simulink model "L400_airframe"  (R2024b)
settings: Solver=FixedStepAuto  StartTime=0  StopTime=10  FixedStep=5/1000  RelTol=1e-3
values from neighbouring files (symbols this model uses):
  db =     [L400_airframe_data.mat]
undefined symbols (not defined in the file or in its folder): lambda
libraries: aerolibconvert2 x16, simulink x6, matrix_library x4, aerolibactuator x2, shared6dof x1, aerolibtransform2 x1
(part 4 of 4)

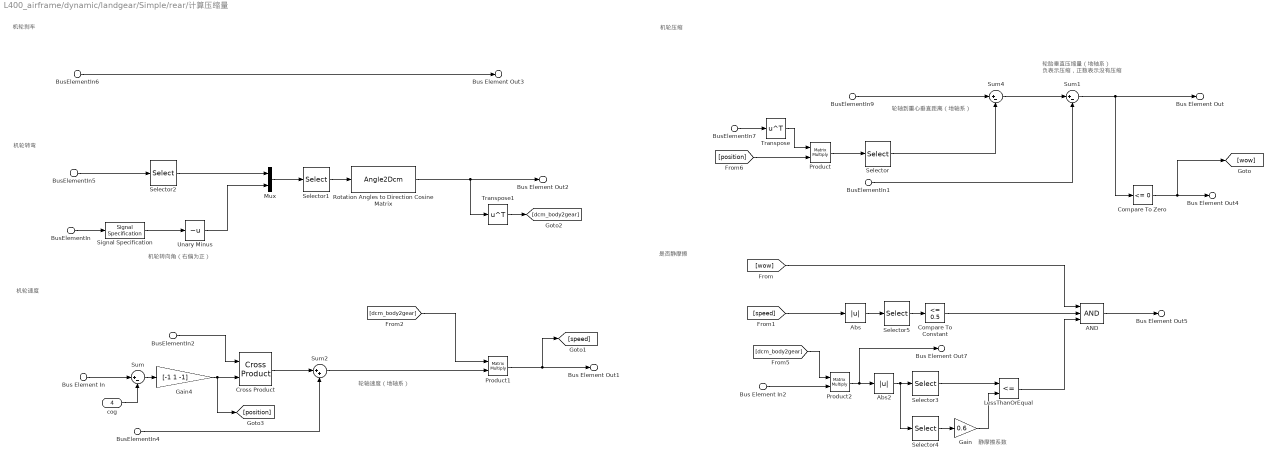
== system L400_airframe/dynamic/landgear/Simple/rear/计算压缩量 ==
  note: 静摩擦系数
  note: 机轮刹车
  note: 是否静摩擦
  note: 机轮速度
  note: 机轮转弯
  note: 机轮压缩
  note: 机轮转向角（右偏为正）
  note: 轮胎垂直压缩量（地轴系）
      | 负表示压缩，正数表示没有压缩
  note: 轮轴到重心垂直距离（地轴系）
  note: 轮轴速度（地轴系）
  BusElementIn : Inport  PortName=cmd  Element=DWheel
  BusElementIn6 : Inport  PortName=cmd  Element=DBrake
  BusElementIn7 : Inport  Port=2  PortName=state  Element=aircraft.attitude.Rbe
  BusElementIn2 : Inport  Port=2  PortName=state  Element=aircraft.attitude.p_q_r
  BusElementIn5 : Inport  Port=2  PortName=state  Element=aircraft.attitude.phi_theta_psi
  BusElementIn4 : Inport  Port=2  PortName=state  Element=aircraft.position.vx_vy_vz
  BusElementIn9 : Inport  Port=2  PortName=state  Element=aircraft.position.alt
  BusElementIn1 : Inport  Port=2  PortName=state  Element=environ.terrain.hground
  Bus Element In : Inport  Port=3  PortName=param  Element=position
  Bus Element In2 : Inport  Port=3  PortName=param  Element=reaction
  cog : Inport  Port=4
  AND : Logic  Inputs=3  IconShape=distinctive  AllPortsSameDT=off  OutDataTypeStr=boolean
  Abs : Abs  SaturateOnIntegerOverflow=off
  Abs2 : Abs  SaturateOnIntegerOverflow=off
  Compare To Constant : simulink/Logic and Bit Operations/Compare To Constant  relop=<=  const=0.5  OutDataTypeStr=boolean
  Compare To Zero : simulink/Logic and Bit Operations/Compare To Zero  relop=<=  OutDataTypeStr=boolean
  Cross Product : matrix_library/Cross Product
  Gain : Gain  Gain=0.6
  Gain4 : Gain  Gain=[-1 1 -1]
  LessThanOrEqual : RelationalOperator  Operator=<=  OutDataTypeStr=boolean  RndMeth=Simplest  InputSameDT=off
  Mux : Mux  Inputs=2
  Product : Product  Multiplication=Matrix(*)
  Product1 : Product  Multiplication=Matrix(*)
  Product2 : Product  Multiplication=Matrix(*)
  Rotation Angles to Direction Cosine Matrix : Angle2Dcm
      settings: AttributesFormatString=Rotation Order: %<rotationOrder>
  Selector : Selector  InputPortWidth=3  IndexOptions=Index vector (dialog)  Indices=3  OutputSizes=1
  Selector1 : Selector  InputPortWidth=3  IndexOptions=Index vector (dialog)  Indices=[3 2 1]  OutputSizes=1
  Selector2 : Selector  InputPortWidth=3  IndexOptions=Index vector (dialog)  Indices=[1 2]  OutputSizes=1
  Selector3 : Selector  InputPortWidth=3  IndexOptions=Index vector (dialog)  Indices=[1 2]  OutputSizes=1
  Selector4 : Selector  InputPortWidth=3  IndexOptions=Index vector (dialog)  Indices=3  OutputSizes=1
  Selector5 : Selector  InputPortWidth=3  IndexOptions=Index vector (dialog)  Indices=[1 2]  OutputSizes=1
  Signal Specification : SignalSpecification  Unit=rad
  Sum : Sum  Inputs=|+-
  Sum1 : Sum  Inputs=|+-
  Sum2 : Sum  Inputs=|++
  Sum4 : Sum  Inputs=|+-
  Transpose : Math  Operator=transpose
  Transpose1 : Math  Operator=transpose
  Unary Minus : UnaryMinus
  Bus Element Out : Outport  PortName=gear  Element=cmprs
  Bus Element Out1 : Outport  PortName=gear  Element=speed
  Bus Element Out2 : Outport  PortName=gear  Element=dcm_gear2body
  Bus Element Out3 : Outport  PortName=gear  Element=lambda
  Bus Element Out4 : Outport  PortName=gear  Element=wow
  Bus Element Out5 : Outport  PortName=gear  Element=istatic
  Bus Element Out7 : Outport  PortName=gear  Element=reaction
  wires:
  BusElementIn/1 -> Signal Specification/1
  Signal Specification/1 -> Unary Minus/1
  Mux/1 -> Selector1/1
  Product1/1 -> [speed], Bus Element Out1/1
  Compare To Zero/1 -> [wow], Bus Element Out4/1
  BusElementIn7/1 -> Transpose/1
  Sum4/1 -> Sum1/1
  Sum2/1 -> Product1/2
  Product/1 -> Selector/1
  BusElementIn9/1 -> Sum4/1
  Selector/1 -> Sum4/2
  Transpose/1 -> Product/1
  [position] -> Product/2
  BusElementIn4/1 -> Sum2/2
  Sum1/1 -> Compare To Zero/1, Bus Element Out/1
  Cross Product/1 -> Sum2/1
  BusElementIn1/1 -> Sum1/2
  BusElementIn2/1 -> Cross Product/1
  Selector1/1 -> Rotation Angles to Direction Cosine Matrix/1
  Rotation Angles to Direction Cosine Matrix/1 -> Bus Element Out2/1, Transpose1/1
  Bus Element In2/1 -> Product2/2
  [dcm_body2gear] -> Product1/1
  Compare To Constant/1 -> AND/2
  Abs/1 -> Selector5/1
  [wow] -> AND/1
  [speed] -> Abs/1
  Transpose1/1 -> [dcm_body2gear]
  [dcm_body2gear] -> Product2/1
  Product2/1 -> Abs2/1, Bus Element Out7/1
  Selector4/1 -> Gain/1
  Gain/1 -> LessThanOrEqual/2
  LessThanOrEqual/1 -> AND/3
  AND/1 -> Bus Element Out5/1
  Bus Element In/1 -> Sum/1
  cog/1 -> Sum/2
  Sum/1 -> Gain4/1
  Gain4/1 -> [position], Cross Product/2
  BusElementIn5/1 -> Selector2/1
  Selector2/1 -> Mux/1
  Unary Minus/1 -> Mux/2
  Abs2/1 -> Selector4/1, Selector3/1
  Selector3/1 -> LessThanOrEqual/1
  Selector5/1 -> Compare To Constant/1
  BusElementIn6/1 -> Bus Element Out3/1

== system L400_airframe/dynamic/landgear/Simple/right/侧向摩擦力 ==
  note: % Compute the sideforce coefficients using Pacejka's Magic Formula.
      | %
      | % y(x) = D sin {C arctan [Bx - E(Bx - arctan Bx)]}
      | %
      | % Where: B = Stiffness Factor (0.06, here)
      | % C = Shape Factor (2.8, here)
      | % D = Peak Factor (0.8, here)
      | % E = Curvature Factor (1.03, here)
  Bus Element In3 : Inport  PortName=gear  Element=speed
  Bus Element In2 : Inport  PortName=gear  Element=istatic
  Bus Element In1 : Inport  PortName=gear  Element=reaction
  |Fz| : Inport  Port=2
  Angle Conversion : aerolibconvert2/Angle Conversion  IU=rad  OU=deg
  Atan : Trigonometry  Operator=atan
  Atan1 : Trigonometry  Operator=atan
  Atan2 : Trigonometry  Operator=atan2
  Atan3 : Trigonometry
  Demux : Demux  Outputs=2
  Gain : Gain  Gain=0.06
  Gain1 : Gain  Gain=1.03
  Gain2 : Gain  Gain=2.8
  Gain3 : Gain  Gain=0.8
  Product : Product
  Selector1 : Selector  InputPortWidth=3  IndexOptions=Index vector (dialog)  Indices=[2, 1]  OutputSizes=1
  Selector2 : Selector  InputPortWidth=2  IndexOptions=Index vector (dialog)  Indices=2  OutputSizes=1
  Selector3 : Selector  InputPortWidth=3  IndexOptions=Index vector (dialog)  Indices=2  OutputSizes=1
  Sum : Sum  Inputs=+-|
  Sum1 : Sum  Inputs=|+-
  Switch : Switch  Criteria=u2 > Threshold  Threshold=0.5  SaturateOnIntegerOverflow=off  InputSameDT=off
  Unary Minus : UnaryMinus
  Fy : Outport
  wires:
  Switch/1 -> Fy/1
  Bus Element In3/1 -> Selector1/1
  Demux/2 -> Atan2/2
  Selector1/1 -> Demux/1
  Demux/1 -> Atan2/1
  Selector2/1 -> Switch/2
  Bus Element In2/1 -> Selector2/1
  Bus Element In1/1 -> Selector3/1
  Selector3/1 -> Switch/1
  Product/1 -> Unary Minus/1
  Gain/1 -> Sum/1, Sum1/1, Atan/1
  Atan/1 -> Sum/2
  Gain2/1 -> Atan3/1
  Sum1/1 -> Atan1/1
  Sum/1 -> Gain1/1
  Atan1/1 -> Gain2/1
  Gain1/1 -> Sum1/2
  Atan2/1 -> Angle Conversion/1
  Atan3/1 -> Gain3/1
  Angle Conversion/1 -> Gain/1
  Gain3/1 -> Product/1
  |Fz|/1 -> Product/2
  Unary Minus/1 -> Switch/3

== system L400_airframe/dynamic/landgear/Simple/right/地面支反力 ==
  note: 阻尼力
  note: 起落架缓冲器所提供的缓冲力是起落架提供给飞机支反力的主要组成部分，主要由随压缩行程变化的弹簧力、随压缩速率变化的阻尼力以及缓冲器内部有相对运动而产生的滑动摩擦力组成。
  note: 弹簧力
  note: 摩擦力
  note: 轮胎支反力
  note: 弹簧力刚度系数可以大概如下估算：
      | 无人机重力8000N，一共3个轮胎，假设平衡时轮胎压缩1cm，那么
      | K = 8000/3/0.01 ≈ 2.5e5
      | 弹簧系数一定不要打了，否则很容易发散
  Bus Element In1 : Inport  PortName=gear  Element=cmprs
  Bus Element In2 : Inport  PortName=gear  Element=speed
  Gain2 : Gain  Gain=1e5
  Gain3 : Gain  Gain=-1e3
  Gain7 : Gain  Gain=0
  Saturation : Saturate  UpperLimit=0  LowerLimit=-1
  Selector3 : Selector  InputPortWidth=3  IndexOptions=Index vector (dialog)  Indices=3  OutputSizes=1
  Sign : Signum
  Sum3 : Sum  Inputs=3
  Fz : Outport
  wires:
  Gain7/1 -> Sum3/3
  Bus Element In2/1 -> Selector3/1
  Sum3/1 -> Fz/1
  Sign/1 -> Gain7/1
  Saturation/1 -> Gain2/1
  Selector3/1 -> Sign/1, Gain3/1
  Gain3/1 -> Sum3/2
  Gain2/1 -> Sum3/1
  Bus Element In1/1 -> Saturation/1

== system L400_airframe/dynamic/landgear/Simple/right/纵向摩擦力 ==
  note: 刹车摩擦系数，采用轮胎的魔术公式
      | μ = D sin(C*atan(Bλ))
      | 其中λ是滑移率
  note: 滚动摩擦系数
  BusElementIn3 : Inport  PortName=gear  Element=lambda
  BusElementIn2 : Inport  PortName=gear  Element=istatic
  BusElementIn4 : Inport  PortName=gear  Element=reaction
  BusElementIn1 : Inport  PortName=gear  Element=speed
  |Fz| : Inport  Port=2
  B : Gain  Gain=14.032
  C : Gain  Gain=1.5344
  Constant : Constant  Value=0.02
  D : Gain  Gain=0.8
  Product : Product
  Product1 : Product
  Selector : Selector  InputPortWidth=3  IndexOptions=Index vector (dialog)  Indices=1  OutputSizes=1
  Selector1 : Selector  InputPortWidth=2  IndexOptions=Index vector (dialog)  Indices=1  OutputSizes=1
  Selector5 : Selector  InputPortWidth=3  IndexOptions=Index vector (dialog)  Indices=1  OutputSizes=1
  Sign : Signum
  Sin : Trigonometry
  Sin1 : Trigonometry  Operator=atan
  Sum : Sum  Inputs=|++
  Switch : Switch  Criteria=u2 > Threshold  Threshold=0.5  SaturateOnIntegerOverflow=off  InputSameDT=off
  Unary Minus : UnaryMinus
  Fx : Outport
  wires:
  BusElementIn3/1 -> B/1
  Sin/1 -> D/1
  B/1 -> Sin1/1
  Sin1/1 -> C/1
  C/1 -> Sin/1
  Constant/1 -> Product1/1
  D/1 -> Sum/1
  BusElementIn4/1 -> Selector5/1
  Switch/1 -> Fx/1
  Selector5/1 -> Switch/1
  BusElementIn2/1 -> Selector1/1
  Selector1/1 -> Switch/2
  BusElementIn1/1 -> Selector/1
  Selector/1 -> Sign/1
  Sign/1 -> Product1/2
  Product1/1 -> Sum/2
  Product/1 -> Unary Minus/1
  |Fz|/1 -> Product/2
  Unary Minus/1 -> Switch/3
  Sum/1 -> Product/1

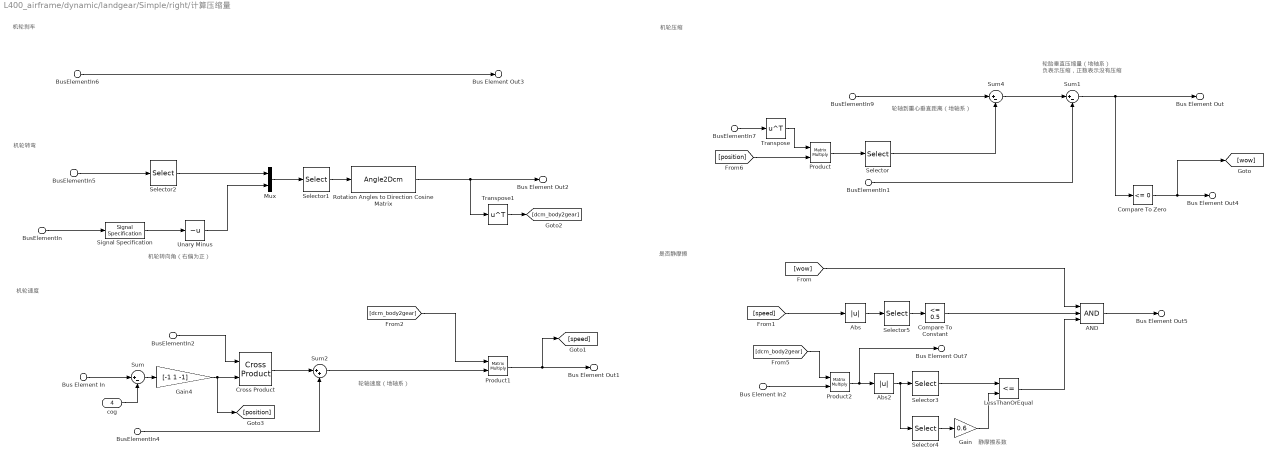
== system L400_airframe/dynamic/landgear/Simple/right/计算压缩量 ==
  note: 静摩擦系数
  note: 机轮刹车
  note: 是否静摩擦
  note: 机轮速度
  note: 机轮转弯
  note: 机轮压缩
  note: 机轮转向角（右偏为正）
  note: 轮胎垂直压缩量（地轴系）
      | 负表示压缩，正数表示没有压缩
  note: 轮轴到重心垂直距离（地轴系）
  note: 轮轴速度（地轴系）
  BusElementIn : Inport  PortName=cmd  Element=DWheel
  BusElementIn6 : Inport  PortName=cmd  Element=DBrake
  BusElementIn7 : Inport  Port=2  PortName=state  Element=aircraft.attitude.Rbe
  BusElementIn2 : Inport  Port=2  PortName=state  Element=aircraft.attitude.p_q_r
  BusElementIn5 : Inport  Port=2  PortName=state  Element=aircraft.attitude.phi_theta_psi
  BusElementIn4 : Inport  Port=2  PortName=state  Element=aircraft.position.vx_vy_vz
  BusElementIn9 : Inport  Port=2  PortName=state  Element=aircraft.position.alt
  BusElementIn1 : Inport  Port=2  PortName=state  Element=environ.terrain.hground
  Bus Element In : Inport  Port=3  PortName=param  Element=position
  Bus Element In2 : Inport  Port=3  PortName=param  Element=reaction
  cog : Inport  Port=4
  AND : Logic  Inputs=3  IconShape=distinctive  AllPortsSameDT=off  OutDataTypeStr=boolean
  Abs : Abs  SaturateOnIntegerOverflow=off
  Abs2 : Abs  SaturateOnIntegerOverflow=off
  Compare To Constant : simulink/Logic and Bit Operations/Compare To Constant  relop=<=  const=0.5  OutDataTypeStr=boolean
  Compare To Zero : simulink/Logic and Bit Operations/Compare To Zero  relop=<=  OutDataTypeStr=boolean
  Cross Product : matrix_library/Cross Product
  Gain : Gain  Gain=0.6
  Gain4 : Gain  Gain=[-1 1 -1]
  LessThanOrEqual : RelationalOperator  Operator=<=  OutDataTypeStr=boolean  RndMeth=Simplest  InputSameDT=off
  Mux : Mux  Inputs=2
  Product : Product  Multiplication=Matrix(*)
  Product1 : Product  Multiplication=Matrix(*)
  Product2 : Product  Multiplication=Matrix(*)
  Rotation Angles to Direction Cosine Matrix : Angle2Dcm
      settings: AttributesFormatString=Rotation Order: %<rotationOrder>
  Selector : Selector  InputPortWidth=3  IndexOptions=Index vector (dialog)  Indices=3  OutputSizes=1
  Selector1 : Selector  InputPortWidth=3  IndexOptions=Index vector (dialog)  Indices=[3 2 1]  OutputSizes=1
  Selector2 : Selector  InputPortWidth=3  IndexOptions=Index vector (dialog)  Indices=[1 2]  OutputSizes=1
  Selector3 : Selector  InputPortWidth=3  IndexOptions=Index vector (dialog)  Indices=[1 2]  OutputSizes=1
  Selector4 : Selector  InputPortWidth=3  IndexOptions=Index vector (dialog)  Indices=3  OutputSizes=1
  Selector5 : Selector  InputPortWidth=3  IndexOptions=Index vector (dialog)  Indices=[1 2]  OutputSizes=1
  Signal Specification : SignalSpecification  Unit=rad
  Sum : Sum  Inputs=|+-
  Sum1 : Sum  Inputs=|+-
  Sum2 : Sum  Inputs=|++
  Sum4 : Sum  Inputs=|+-
  Transpose : Math  Operator=transpose
  Transpose1 : Math  Operator=transpose
  Unary Minus : UnaryMinus
  Bus Element Out : Outport  PortName=gear  Element=cmprs
  Bus Element Out1 : Outport  PortName=gear  Element=speed
  Bus Element Out2 : Outport  PortName=gear  Element=dcm_gear2body
  Bus Element Out3 : Outport  PortName=gear  Element=lambda
  Bus Element Out4 : Outport  PortName=gear  Element=wow
  Bus Element Out5 : Outport  PortName=gear  Element=istatic
  Bus Element Out7 : Outport  PortName=gear  Element=reaction
  wires:
  BusElementIn/1 -> Signal Specification/1
  Signal Specification/1 -> Unary Minus/1
  Mux/1 -> Selector1/1
  Product1/1 -> [speed], Bus Element Out1/1
  Compare To Zero/1 -> [wow], Bus Element Out4/1
  BusElementIn7/1 -> Transpose/1
  Sum4/1 -> Sum1/1
  Sum2/1 -> Product1/2
  Product/1 -> Selector/1
  BusElementIn9/1 -> Sum4/1
  Selector/1 -> Sum4/2
  Transpose/1 -> Product/1
  [position] -> Product/2
  BusElementIn4/1 -> Sum2/2
  Sum1/1 -> Compare To Zero/1, Bus Element Out/1
  Cross Product/1 -> Sum2/1
  BusElementIn1/1 -> Sum1/2
  BusElementIn2/1 -> Cross Product/1
  Selector1/1 -> Rotation Angles to Direction Cosine Matrix/1
  Rotation Angles to Direction Cosine Matrix/1 -> Bus Element Out2/1, Transpose1/1
  Bus Element In2/1 -> Product2/2
  [dcm_body2gear] -> Product1/1
  Compare To Constant/1 -> AND/2
  Abs/1 -> Selector5/1
  [wow] -> AND/1
  [speed] -> Abs/1
  Transpose1/1 -> [dcm_body2gear]
  [dcm_body2gear] -> Product2/1
  Product2/1 -> Abs2/1, Bus Element Out7/1
  Selector4/1 -> Gain/1
  Gain/1 -> LessThanOrEqual/2
  LessThanOrEqual/1 -> AND/3
  AND/1 -> Bus Element Out5/1
  Bus Element In/1 -> Sum/1
  cog/1 -> Sum/2
  Sum/1 -> Gain4/1
  Gain4/1 -> [position], Cross Product/2
  BusElementIn5/1 -> Selector2/1
  Selector2/1 -> Mux/1
  Unary Minus/1 -> Mux/2
  Abs2/1 -> Selector4/1, Selector3/1
  Selector3/1 -> LessThanOrEqual/1
  Selector5/1 -> Compare To Constant/1
  BusElementIn6/1 -> Bus Element Out3/1

== system L400_airframe/dynamic/aerodynamic/aerodynamics/If Action Subsystem/CY/Subsystem ==
  alpha : Inport  Unit=deg
  beta : Inport  Port=2  Unit=deg
  H : Inport  Port=3
  TC : Inport  Port=4
  DFLI : Inport  Port=5
  DFLO : Inport  Port=6
  DFRI : Inport  Port=7
  DFRO : Inport  Port=8
  DAL : Inport  Port=9
  DAR : Inport  Port=10
  DEL : Inport  Port=11
  DEM : Inport  Port=12
  DER : Inport  Port=13
  DR : Inport  Port=14
  2-D Lookup Table1 : Lookup_n-D  LookupTableObject=''  BreakpointsForDimension1=db.aerody.VDF  BreakpointsForDimension2=db.aerody.VALPHA  BreakpointsForDimension1FirstPoint=10  BreakpointsForDimension2FirstPoint=10  BreakpointsForDimension1Spacing=12  BreakpointsForDimension2Spacing=12  IndexSearchMethod=Linear search  BeginIndexSearchUsingPreviousIndexResult=on  Table=db.aerody.CYDFLI  ExtrapMethod=Clip  DiagnosticForOutOfRangeInput=Warning  InternalRulePriority=Speed  RndMeth=Simplest
      settings: InputPortMap=u0,u1
  2-D Lookup Table10 : Lookup_n-D  LookupTableObject=''  BreakpointsForDimension1=db.aerody.VDE  BreakpointsForDimension2=db.aerody.VALPHA  BreakpointsForDimension1FirstPoint=10  BreakpointsForDimension2FirstPoint=10  BreakpointsForDimension1Spacing=12  BreakpointsForDimension2Spacing=12  IndexSearchMethod=Linear search  BeginIndexSearchUsingPreviousIndexResult=on  Table=db.aerody.CYDER  ExtrapMethod=Clip  DiagnosticForOutOfRangeInput=Warning  InternalRulePriority=Speed  RndMeth=Simplest
      settings: InputPortMap=u0,u1
  2-D Lookup Table12 : Lookup_n-D  LookupTableObject=''  BreakpointsForDimension1=db.aerody.VDR  BreakpointsForDimension2=db.aerody.VALPHA  BreakpointsForDimension1FirstPoint=10  BreakpointsForDimension2FirstPoint=10  BreakpointsForDimension1Spacing=12  BreakpointsForDimension2Spacing=12  IndexSearchMethod=Linear search  BeginIndexSearchUsingPreviousIndexResult=on  Table=db.aerody.CYDR  ExtrapMethod=Clip  DiagnosticForOutOfRangeInput=Warning  InternalRulePriority=Speed  RndMeth=Simplest
      settings: InputPortMap=u0,u1
  2-D Lookup Table13 : Lookup_n-D  NumberOfTableDimensions=3  LookupTableObject=''  BreakpointsForDimension1=db.aerody.VDR  BreakpointsForDimension2=db.aerody.VALPHA  BreakpointsForDimension3=db.aerody.VBETA  BreakpointsForDimension1FirstPoint=10  BreakpointsForDimension2FirstPoint=10  BreakpointsForDimension1Spacing=12  BreakpointsForDimension2Spacing=12  IndexSearchMethod=Linear search  BeginIndexSearchUsingPreviousIndexResult=on  Table=db.aerody.CYDRBETA  ExtrapMethod=Clip  DiagnosticForOutOfRangeInput=Warning  InternalRulePriority=Speed  RndMeth=Simplest
      settings: InputPortMap=u0,u1,u2
  2-D Lookup Table16 : Lookup_n-D  NumberOfTableDimensions=3  LookupTableObject=''  BreakpointsForDimension1=db.aerody.VH  BreakpointsForDimension2=db.aerody.VALPHA  BreakpointsForDimension3=db.aerody.VDF  BreakpointsForDimension1FirstPoint=10  BreakpointsForDimension2FirstPoint=10  BreakpointsForDimension1Spacing=12  BreakpointsForDimension2Spacing=12  IndexSearchMethod=Linear search  BeginIndexSearchUsingPreviousIndexResult=on  Table=db.aerody.CYHDFLI  ExtrapMethod=Clip  DiagnosticForOutOfRangeInput=Warning  InternalRulePriority=Speed  RndMeth=Simplest
      settings: InputPortMap=u0,u1,u2
  2-D Lookup Table17 : Lookup_n-D  NumberOfTableDimensions=3  LookupTableObject=''  BreakpointsForDimension1=db.aerody.VH  BreakpointsForDimension2=db.aerody.VALPHA  BreakpointsForDimension3=db.aerody.VDF  BreakpointsForDimension1FirstPoint=10  BreakpointsForDimension2FirstPoint=10  BreakpointsForDimension1Spacing=12  BreakpointsForDimension2Spacing=12  IndexSearchMethod=Linear search  BeginIndexSearchUsingPreviousIndexResult=on  Table=db.aerody.CYHDFLO  ExtrapMethod=Clip  DiagnosticForOutOfRangeInput=Warning  InternalRulePriority=Speed  RndMeth=Simplest
      settings: InputPortMap=u0,u1,u2
  2-D Lookup Table18 : Lookup_n-D  NumberOfTableDimensions=3  LookupTableObject=''  BreakpointsForDimension1=db.aerody.VH  BreakpointsForDimension2=db.aerody.VALPHA  BreakpointsForDimension3=db.aerody.VDF  BreakpointsForDimension1FirstPoint=10  BreakpointsForDimension2FirstPoint=10  BreakpointsForDimension1Spacing=12  BreakpointsForDimension2Spacing=12  IndexSearchMethod=Linear search  BeginIndexSearchUsingPreviousIndexResult=on  Table=db.aerody.CYHDFRI  ExtrapMethod=Clip  DiagnosticForOutOfRangeInput=Warning  InternalRulePriority=Speed  RndMeth=Simplest
      settings: InputPortMap=u0,u1,u2
  2-D Lookup Table19 : Lookup_n-D  NumberOfTableDimensions=3  LookupTableObject=''  BreakpointsForDimension1=db.aerody.VH  BreakpointsForDimension2=db.aerody.VALPHA  BreakpointsForDimension3=db.aerody.VDF  BreakpointsForDimension1FirstPoint=10  BreakpointsForDimension2FirstPoint=10  BreakpointsForDimension1Spacing=12  BreakpointsForDimension2Spacing=12  IndexSearchMethod=Linear search  BeginIndexSearchUsingPreviousIndexResult=on  Table=db.aerody.CYHDFRO  ExtrapMethod=Clip  DiagnosticForOutOfRangeInput=Warning  InternalRulePriority=Speed  RndMeth=Simplest
      settings: InputPortMap=u0,u1,u2
  2-D Lookup Table2 : Lookup_n-D  LookupTableObject=''  BreakpointsForDimension1=db.aerody.VDF  BreakpointsForDimension2=db.aerody.VALPHA  BreakpointsForDimension1FirstPoint=10  BreakpointsForDimension2FirstPoint=10  BreakpointsForDimension1Spacing=12  BreakpointsForDimension2Spacing=12  IndexSearchMethod=Linear search  BeginIndexSearchUsingPreviousIndexResult=on  Table=db.aerody.CYDFRI  ExtrapMethod=Clip  DiagnosticForOutOfRangeInput=Warning  InternalRulePriority=Speed  RndMeth=Simplest
      settings: InputPortMap=u0,u1
  2-D Lookup Table20 : Lookup_n-D  LookupTableObject=''  BreakpointsForDimension1=db.aerody.VTC  BreakpointsForDimension2=db.aerody.VALPHA  BreakpointsForDimension1FirstPoint=10  BreakpointsForDimension2FirstPoint=10  BreakpointsForDimension1Spacing=12  BreakpointsForDimension2Spacing=12  IndexSearchMethod=Linear search  BeginIndexSearchUsingPreviousIndexResult=on  Table=db.aerody.CYSS  ExtrapMethod=Clip  DiagnosticForOutOfRangeInput=Warning  InternalRulePriority=Speed  RndMeth=Simplest
      settings: InputPortMap=u0,u1
  2-D Lookup Table3 : Lookup_n-D  LookupTableObject=''  BreakpointsForDimension1=db.aerody.VDF  BreakpointsForDimension2=db.aerody.VALPHA  BreakpointsForDimension1FirstPoint=10  BreakpointsForDimension2FirstPoint=10  BreakpointsForDimension1Spacing=12  BreakpointsForDimension2Spacing=12  IndexSearchMethod=Linear search  BeginIndexSearchUsingPreviousIndexResult=on  Table=db.aerody.CYDFRO  ExtrapMethod=Clip  DiagnosticForOutOfRangeInput=Warning  InternalRulePriority=Speed  RndMeth=Simplest
      settings: InputPortMap=u0,u1
  2-D Lookup Table4 : Lookup_n-D  LookupTableObject=''  BreakpointsForDimension1=db.aerody.VDA  BreakpointsForDimension2=db.aerody.VALPHA  BreakpointsForDimension1FirstPoint=10  BreakpointsForDimension2FirstPoint=10  BreakpointsForDimension1Spacing=12  BreakpointsForDimension2Spacing=12  IndexSearchMethod=Linear search  BeginIndexSearchUsingPreviousIndexResult=on  Table=db.aerody.CYDAL  ExtrapMethod=Clip  DiagnosticForOutOfRangeInput=Warning  InternalRulePriority=Speed  RndMeth=Simplest
      settings: InputPortMap=u0,u1
  2-D Lookup Table5 : Lookup_n-D  LookupTableObject=''  BreakpointsForDimension1=db.aerody.VDA  BreakpointsForDimension2=db.aerody.VALPHA  BreakpointsForDimension1FirstPoint=10  BreakpointsForDimension2FirstPoint=10  BreakpointsForDimension1Spacing=12  BreakpointsForDimension2Spacing=12  IndexSearchMethod=Linear search  BeginIndexSearchUsingPreviousIndexResult=on  Table=db.aerody.CYDAR  ExtrapMethod=Clip  DiagnosticForOutOfRangeInput=Warning  InternalRulePriority=Speed  RndMeth=Simplest
      settings: InputPortMap=u0,u1
  2-D Lookup Table6 : Lookup_n-D  LookupTableObject=''  BreakpointsForDimension1=db.aerody.VDF  BreakpointsForDimension2=db.aerody.VALPHA  BreakpointsForDimension1FirstPoint=10  BreakpointsForDimension2FirstPoint=10  BreakpointsForDimension1Spacing=12  BreakpointsForDimension2Spacing=12  IndexSearchMethod=Linear search  BeginIndexSearchUsingPreviousIndexResult=on  Table=db.aerody.CYDFLO  ExtrapMethod=Clip  DiagnosticForOutOfRangeInput=Warning  InternalRulePriority=Speed  RndMeth=Simplest
      settings: InputPortMap=u0,u1
  2-D Lookup Table7 : Lookup_n-D  LookupTableObject=''  BreakpointsForDimension1=db.aerody.VBETA  BreakpointsForDimension2=db.aerody.VALPHA  BreakpointsForDimension1FirstPoint=10  BreakpointsForDimension2FirstPoint=10  BreakpointsForDimension1Spacing=12  BreakpointsForDimension2Spacing=12  IndexSearchMethod=Linear search  BeginIndexSearchUsingPreviousIndexResult=on  Table=db.aerody.CYBETA  ExtrapMethod=Clip  DiagnosticForOutOfRangeInput=Warning  InternalRulePriority=Speed  RndMeth=Simplest
      settings: InputPortMap=u0,u1
  2-D Lookup Table8 : Lookup_n-D  LookupTableObject=''  BreakpointsForDimension1=db.aerody.VDE  BreakpointsForDimension2=db.aerody.VALPHA  BreakpointsForDimension1FirstPoint=10  BreakpointsForDimension2FirstPoint=10  BreakpointsForDimension1Spacing=12  BreakpointsForDimension2Spacing=12  IndexSearchMethod=Linear search  BeginIndexSearchUsingPreviousIndexResult=on  Table=db.aerody.CYDEL  ExtrapMethod=Clip  DiagnosticForOutOfRangeInput=Warning  InternalRulePriority=Speed  RndMeth=Simplest
      settings: InputPortMap=u0,u1
  2-D Lookup Table9 : Lookup_n-D  LookupTableObject=''  BreakpointsForDimension1=db.aerody.VDE  BreakpointsForDimension2=db.aerody.VALPHA  BreakpointsForDimension1FirstPoint=10  BreakpointsForDimension2FirstPoint=10  BreakpointsForDimension1Spacing=12  BreakpointsForDimension2Spacing=12  IndexSearchMethod=Linear search  BeginIndexSearchUsingPreviousIndexResult=on  Table=db.aerody.CYDEM  ExtrapMethod=Clip  DiagnosticForOutOfRangeInput=Warning  InternalRulePriority=Speed  RndMeth=Simplest
      settings: InputPortMap=u0,u1
  Gain : Gain
  Saturation : Saturate  UpperLimit=5.8  LowerLimit=0
  Sum : Sum  Inputs=17
  CY : Outport
  wires:
  2-D Lookup Table17/1 -> Sum/3  "CYHDFLO"
  2-D Lookup Table13/1 -> Sum/16  "CYDRBETA"
  2-D Lookup Table1/1 -> Sum/6
  alpha/1 -> 2-D Lookup Table7/2, 2-D Lookup Table20/2, 2-D Lookup Table16/2, 2-D Lookup Table17/2, 2-D Lookup Table18/2, 2-D Lookup Table19/2, 2-D Lookup Table1/2, 2-D Lookup Table6/2, 2-D Lookup Table2/2, 2-D Lookup Table3/2, 2-D Lookup Table4/2, 2-D Lookup Table5/2, 2-D Lookup Table8/2, 2-D Lookup Table9/2, 2-D Lookup Table10/2, 2-D Lookup Table12/2, 2-D Lookup Table13/2
  beta/1 -> 2-D Lookup Table7/1, 2-D Lookup Table13/3
  2-D Lookup Table20/1 -> Sum/1  "CYSS"
  2-D Lookup Table7/1 -> Sum/17  "CYBETA"
  2-D Lookup Table12/1 -> Sum/15  "CYDR"
  2-D Lookup Table6/1 -> Sum/7  "CYDFLI"
  DFRI/1 -> 2-D Lookup Table18/3, 2-D Lookup Table2/1
  2-D Lookup Table2/1 -> Sum/8  "CYDFRI"
  DFRO/1 -> 2-D Lookup Table19/3, 2-D Lookup Table3/1
  DFLI/1 -> 2-D Lookup Table16/3, 2-D Lookup Table1/1
  2-D Lookup Table9/1 -> Sum/13  "CYDEM"
  2-D Lookup Table16/1 -> Sum/2  "CYHDFLI"
  Sum/1 -> Gain/1  "CY1"
  DFLO/1 -> 2-D Lookup Table6/1, 2-D Lookup Table17/3
  2-D Lookup Table8/1 -> Sum/12  "CYDEL"
  2-D Lookup Table19/1 -> Sum/5  "CYHDFRO"
  Gain/1 -> CY/1  "CY"
  2-D Lookup Table5/1 -> Sum/11  "CYDAR"
  H/1 -> Saturation/1
  2-D Lookup Table10/1 -> Sum/14  "CYDER"
  2-D Lookup Table4/1 -> Sum/10  "CYDAL"
  2-D Lookup Table18/1 -> Sum/4  "CYHDFRI"
  DR/1 -> 2-D Lookup Table12/1, 2-D Lookup Table13/1
  DAL/1 -> 2-D Lookup Table4/1
  2-D Lookup Table3/1 -> Sum/9  "CYDFRO"
  DAR/1 -> 2-D Lookup Table5/1
  DER/1 -> 2-D Lookup Table10/1
  TC/1 -> 2-D Lookup Table20/1
  DEL/1 -> 2-D Lookup Table8/1
  DEM/1 -> 2-D Lookup Table9/1
  Saturation/1 -> 2-D Lookup Table19/1, 2-D Lookup Table18/1, 2-D Lookup Table17/1, 2-D Lookup Table16/1

== matlab function L400_airframe/dynamic/landgear/Simple/ground static friction/MATLAB Function ==
  data: Fxyz input; Fstatic output; Mxyz input; POS input; COG input
function Fstatic = calc_static_ground_reaction(Fxyz, Mxyz, POS, COG)
% Fxyz，除了起落架之外总外力
% Mxyz，除了起落架之外的总力矩
% POS， 起落架的安装位置（构型系），每列一个
% COG，重心坐标（构型系）

% 起落架的个数
ngear = size(POS, 2);

% 力平衡方程
AF = repmat(eye(3),   1, ngear);
bF = -Fxyz(:);

% 力矩平衡方程
AM = repmat(zeros(3), 1, ngear);
bM = -Mxyz(:);
for i = 0:ngear-1
    % 将起落架位置转换到重心坐标系
    pos = (POS(:, i+1) - COG(:)) .* [-1; 1; -1];
    AM(:, 3*i+1:3*i+3) = get_cross_mat(pos);
end

% 通过伪逆求支反力
A= [AF; AM];
b= [bF; bM];
Fstatic = reshape(A\b, 3, ngear);
end

function m = get_cross_mat(v)
x = v(1);
y = v(2);
z = v(3);
m = [
    0, -z,  y
    z,  0, -x
    -y, x,  0
    ];
end

== matlab function L400_airframe/dynamic/landgear/Complete/MATLAB Function ==
  data: theta input; y output; varphi input; lambda input; delta input
function y = fcn(theta,varphi,lambda,delta)
y = arctan{(cos(theta)cos(varphi)cos(lambda)-sin(theta)sin(lambda))cos(lambda)+...
    [(sin(theta)cos(lambda)+cos(theta)cos(varphi)sin(lambda))cos(delta)-cos(theta)sin(varphi)sin(delta)]sin(lambda)}/...
    {(cos(theta)cos(varphi)cos(lambda)-sin(theta)sin(lambda))sin(lambda) - ...
    [(sin(theta)cos(lambda)+cos(theta)cos(varphi)sin(lambda))cos(delta)-cos(theta)sin(varphi)sin(delta)]cos(lambda) };
y = u;
